simulink model "attiCon"  (R2015b)
settings: Solver=ode45  StartTime=0.0  StopTime=10.0  RelTol=1e-3
PreLoadFcn:
  | initialize
undefined symbols (not defined in the file or in its folder): ini_q, ini_w
settings Model: Creator=yyas16  LastModifiedBy=yyas16
settings DataIOCC: InitialState=iniAtti  LimitDataPoints=off  SaveFormat=Array
settings DebuggingCC: SolverPrmCheckMsg=warning
settings HardwareCC: ProdBitPerPointer=32  ProdLargestAtomicFloat=None  ProdIntDivRoundTo=Undefined  ProdEndianess=Unspecified  ProdWordSize=32  ProdHWDeviceType=32-bit Generic
settings GRTTargetCC: GeneratePreprocessorConditionals=Disable all
settings ConfigComp: CovModelRefEnable=Off  CovSFcnEnable=off

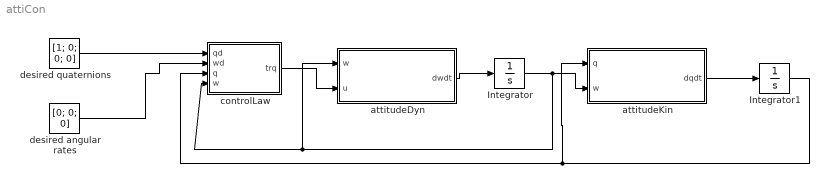
== system attiCon ==
  Integrator : Integrator  InitialCondition=ini_w
  Integrator1 : Integrator  InitialCondition=ini_q
  "attitudeDyn " : MATLAB Function  TreatAsAtomicUnit=on
  attitudeKin : MATLAB Function  TreatAsAtomicUnit=on
  "controlLaw " : MATLAB Function  TreatAsAtomicUnit=on
  desired angular rates : Constant  Value=[0; 0; 0]
  desired quaternions : Constant  Value=[1; 0; 0; 0]
  wires:
  "attitudeDyn "/1(dwdt) -> Integrator/1
  "controlLaw "/1(trq) -> "attitudeDyn "/2(u)
  desired quaternions/1 -> "controlLaw "/1(qd)
  desired angular rates/1 -> "controlLaw "/2(wd)
  Integrator/1 -> "controlLaw "/4(w), "attitudeDyn "/1(w), attitudeKin/2(w)
  attitudeKin/1(dqdt) -> Integrator1/1
  Integrator1/1 -> attitudeKin/1(q), "controlLaw "/3(q)

== matlab function attiCon/controlLaw  ==
  data: qd input; trq output; wd input; q input; w input
function trq  = controlLaw(qd, wd, q, w)
%#codegen
q0 = q(1);
q1 = q(2);
q2 = q(3);
q3 = q(4);
qVec = [q1
    q2
    q3];

wx = w(1);
wy = w(2);
wz = w(3);


trq = -w - qVec;

== matlab function attiCon/attitudeDyn  ==
  data: w input; u input; dwdt output; MOI parameter
function dwdt  = attitudeDyn(w, u, MOI)
%#codegen

% rotational motion
wx = w(1);
wy = w(2);
wz = w(3);

wVec = [wx
    wy
    wz];
dwdt = -MOI^(-1) * cross(wVec, (MOI * wVec)) + MOI^(-1) * u;

== matlab function attiCon/attitudeKin ==
  data: q input; w input; dqdt output
function dqdt  = attitudeKin(q, w)
%#codegen

% rotational motion
%--Quaternion-----------------
q0 = q(1);
q1 = q(2);
q2 = q(3);
q3 = q(4);

wx = w(1);
wy = w(2);
wz = w(3);

qMat = 1.0 / 2.0 .* [-q1 -q2 -q3
    q0 -q3 q2
    q3 q0 -q1
    -q2 q1 q0];

wVec = [wx
    wy
    wz];

dqdt = qMat * wVec;
